simulink model "sim_3tank"  (R2023b)
settings: Solver=VariableStepAuto  StartTime=0.0  StopTime=30  RelTol=1e-3
values from neighbouring files (symbols this model uses):
  initial_state = ((maxinitialstate-mininitialstate).*rand(param.nx,1) + mininitialstate)/10    [main_data_generator.m]    (also in main_simulink_3tanks.m = (b-a).*rand(param.nx,1) + a)
  Ts = 0.1    [dataset_sysID_3tanks.mat]    (also in dataset_sysID_3tanks_final.mat; main_data_generator.m = param.Ts; main_simulink_3tanks.m)
libraries: simulink x1, dspsrcs4 x1
settings Model: Creator=danilo  LastModifiedBy=danilo

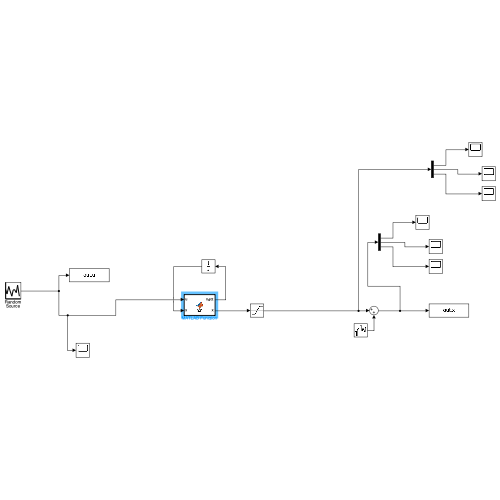
[thumbnail: Simulink's stored preview of the top-level diagram]
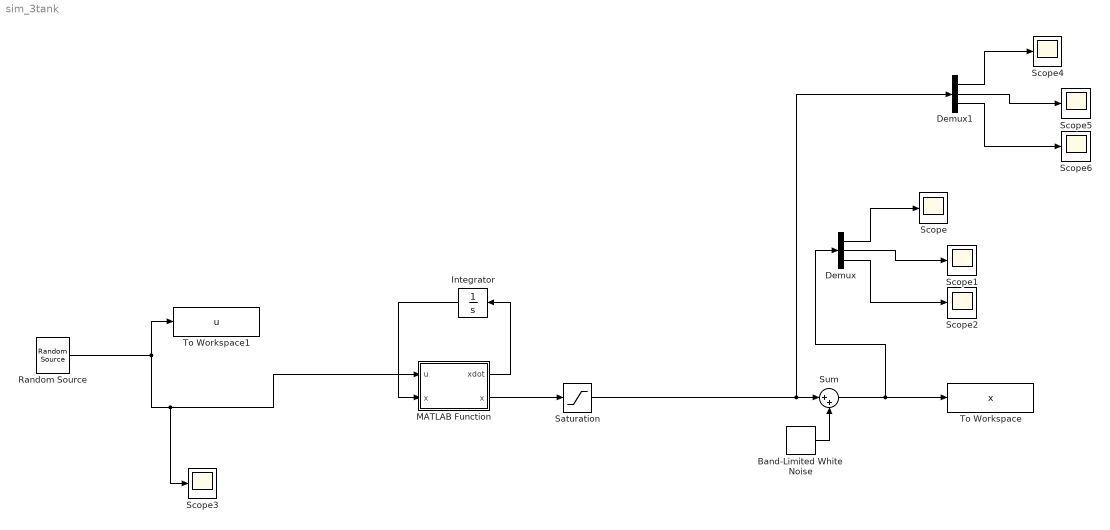
== system sim_3tank ==
  Band-Limited White Noise : simulink/Sources/Band-Limited White Noise  Cov=[0.0001]  Ts=Ts  seed=[23341]
  Demux : Demux  Outputs=3
  Demux1 : Demux  Outputs=3
  Integrator : Integrator  InitialCondition=initial_state
  MATLAB Function : MATLAB Function  TreatAsAtomicUnit=on
  Random Source : dspsrcs4/Random Source  SrcType=Uniform  NormMethod=Ziggurat  CltLength=12  MinVal=10  MaxVal=100  MeanVal=0  VarVal=1  RepMode=Not repeatable  rawSeed=1  IsInherit=off  SampMode=Discrete  SampTime=4  SampFrame=1  DataType=Double  OutComplex=Real  OutputFrames=off
  Saturation : Saturate  UpperLimit=10000  LowerLimit=0
  Scope{,1..6} (7 alike) : Scope
  Sum : Sum  Inputs=|++
  To Workspace : ToWorkspace  VariableName=x  SampleTime=Ts
  To Workspace1 : ToWorkspace  VariableName=u  SampleTime=Ts
  wires:
  Random Source/1 -> Scope3/1, MATLAB Function/1(u), To Workspace1/1
  MATLAB Function/1(xdot) -> Integrator/1
  Integrator/1 -> MATLAB Function/2("x ")
  MATLAB Function/2(x) -> Saturation/1
  Demux/1 -> Scope/1
  Demux/2 -> Scope1/1
  Demux/3 -> Scope2/1
  Sum/1 -> Demux/1, To Workspace/1
  Band-Limited White Noise/1 -> Sum/2
  Demux1/2 -> Scope5/1
  Demux1/1 -> Scope4/1
  Demux1/3 -> Scope6/1
  Saturation/1 -> Demux1/1, Sum/1

== matlab function sim_3tank/MATLAB Function ==
  data: u input; xdot output; x input; x output
function [xdot,x]= fcn(u,x)
param.A1 = 38;% ok
param.A2 = 32;
param.A3 = 21;
param.a1 = 0.05;
param.a2 = 0.03;
param.a3 = 0.06;
param.g = 981;


param.nx = 3;
param.nu = 1;

    if x(1)>=0
        radx1 = (2*param.g*x(1));
    else
        radx1 = 0;
    end
    if x(2)>=0
        radx2 = (2*param.g*x(2));
    else
        radx2 = 0;
    end
    if x(3)>=0
        radx3 = (2*param.g*x(3));
    else
        radx3 = 0;
    end
    xdot = zeros(param.nx,1);

    xdot(1) = -param.a1/param.A1*radx1+0.32*param.a3/param.A1*radx3+50*u(1)/param.A1;    
    xdot(2) = -param.a2/param.A2*radx2+0.23*param.a1/param.A2*radx1;        
    xdot(3) = -param.a3/param.A3*radx3+0.52*param.a2/param.A3*radx2;
